simulink model "pr712"  (R2018b)
settings: Solver=VariableStepAuto  StartTime=0.0  StopTime=20/Rb  RelTol=1e-3
PreLoadFcn:
  | Rb=1e6; % битовая скорость
libraries: commdigbbndpm3 x2, commrandsrc3 x1
settings Model: Creator=Григорий Фокин  LastModifiedBy=Григорий Фокин

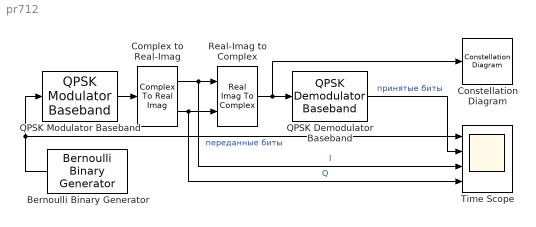
== system pr712 ==
  Bernoulli Binary Generator : commrandsrc3/Bernoulli Binary Generator  ProbabilityOfZero=0.5  SeedSource=Auto  Seed=0  SampleTime=1/Rb  SamplesPerFrame=2  OutputDataType=double  SimulateUsing=Interpreted execution
  Complex to Real-Imag : ComplexToRealImag
  Constellation Diagram : ConstellationDiagram
  QPSK Demodulator Baseband : commdigbbndpm3/QPSK Demodulator Baseband  OutType=Bit  DecType=Hard decision  VarSource=Dialog  Variance=1  Dec=Gray  Ph=pi/4  outDtype1=Inherit via internal rule  outDtype2=Inherit via internal rule  derotateFactorWordLen=16  derotateFactorDataTypeStr=Inherit: Same word length as input  derotateFactorLastDataTypeStr=Inherit: Same word length as input
  QPSK Modulator Baseband : commdigbbndpm3/QPSK Modulator Baseband  InType=Bit  Enc=Gray  Ph=pi/4  outDtype=double  outWordLen=16  outUDDataType=sfix(16)  outFracLenMode=Best precision  outFracLen=15  outDataTypeStr=double  outLastDataTypeStr=double
  Real-Imag to Complex : RealImagToComplex
  Time Scope : Scope  NumInputPorts=4
  wires:
  Bernoulli Binary Generator/1 -> QPSK Modulator Baseband/1, Time Scope/1  "переданные биты"
  QPSK Modulator Baseband/1 -> Complex to Real-Imag/1
  Complex to Real-Imag/1 -> Real-Imag to Complex/1, Time Scope/3  "I"
  Complex to Real-Imag/2 -> Real-Imag to Complex/2, Time Scope/4  "Q"
  Real-Imag to Complex/1 -> QPSK Demodulator Baseband/1, Constellation Diagram/1
  QPSK Demodulator Baseband/1 -> Time Scope/2  "принятые биты"
